simulink model "Project2"  (R2014a)
settings: Solver=ode45  StartTime=0.0  StopTime=10.0  RelTol=1e-3
values from neighbouring files (symbols this model uses):
  A = 3    [Project2_Run.m]
  F = 2    [Project2_Run.m]
  Ti = 0.5    [Project2_Run.m]
libraries: simulink x1
settings Model: Creator=dzr3qn  LastModifiedBy=dzr3qn

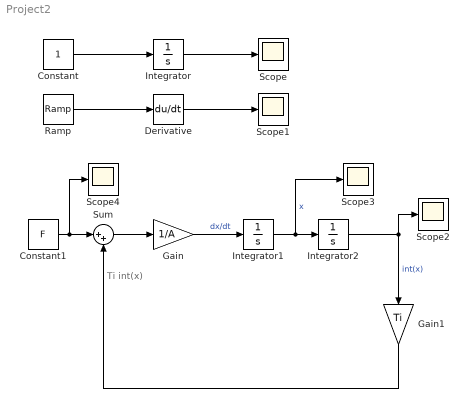
== system Project2 ==
  note: Ti int(x)
  Constant : Constant
  Constant1 : Constant  Value=F
  Derivative : Derivative
  Gain : Gain  Gain=1/A
  Gain1 : Gain  Gain=Ti
  Integrator : Integrator  InitialCondition=2
  Integrator1 : Integrator  InitialCondition=2
  Integrator2 : Integrator  InitialCondition=2
  Ramp : simulink/Sources/Ramp  slope=10  start=0  X0=0
  Scope{,1..4} (5 alike) : Scope
      Scope2 settings: SaveName=ScopeData2
      Scope3 settings: SaveName=ScopeData3
      Scope4 settings: SaveName=ScopeData4
  Sum : Sum  Inputs=|++
  wires:
  Constant/1 -> Integrator/1
  Integrator/1 -> Scope/1
  Ramp/1 -> Derivative/1
  Derivative/1 -> Scope1/1
  Integrator1/1 -> Scope3/1, Integrator2/1  "x"
  Sum/1 -> Gain/1
  Constant1/1 -> Scope4/1, Sum/1
  Gain1/1 -> Sum/2
  Gain/1 -> Integrator1/1  "dx/dt"
  Integrator2/1 -> Scope2/1, Gain1/1  "int(x)"
